simulink library "inp"  (Simulink 7.4)
settings: Solver=ode45  StartTime=0.0  StopTime=10.0  RelTol=1e-3
undefined symbols (not defined in the file): AINP_BrkPedalInterp_X_bar, C_TASK_10MS_S, ENUM_SHIFTER_D, ENUM_SHIFTER_N, ENUM_SHIFTER_P, ENUM_SHIFTER_R, KINP_BonnetCloseVehSpdThre_kph, KINP_EDUCoolantTempFilTm_s, KINP_EDUOilPressureFilTm_s, KINP_EDUOilTempFilTm_s, KINP_EDUSynchDisp_mm, KINP_EDUSynchPosnPWMDC_pct_LowerLimit, KINP_EDUSynchPosnPWMDC_pct_ovrdflg, KINP_EDUSynchPosnPWMDC_pct_ovrdval, KINP_EDUSynchPosnPWMDC_pct_UpperLimit, KINP_ShifterPosConfirmD_s, KINP_ShifterPosConfirmN_s, KINP_ShifterPosConfirmP_s, KINP_ShifterPosConfirmR_s, KINP_SingleAccPedalFltRateLim_pct, KINP_TMSpd2VehSpdSigNeg_rpm, KINP_TMSpd2VehSpdSigPos_rpm, KINP_ValidCheck_EDUSynchPosnPWMDC_dec, KINP_ValidCheck_EDUSynchPosnPWMDC_inc, KINP_ValidCheck_EDUSynchPosnPWMDC_lim, KINP_VehSpdSigKeepThres_kph, KPH2MPS, MIN2SEC, MINP_BrkPedalInterp_pct, MPS2KPH, PI, seat_version_control_block_callbacks, TIRE_RADIUS
libraries: inp_lib x166, hcu_lib x4, simulink x1
(part 7 of 9)

== system inp/INP/INP_20MS/HW_HCU_20ms ==
  BHAL_IN_20ms : Inport
  BSRV_In_ovrdflgs : Inport  Port=2
  BSRV_In_ovrdvals : Inport  Port=3
  Bus Creator : BusCreator  Inputs=2
  Bus Selector18 : BusSelector  OutputSignals=VSRV_EDUOilPressureIn_bar_ovrdval
  Bus Selector20 : BusSelector  OutputSignals=VSRV_EDUOilPressureIn_bar_ovrdflg
  Bus Selector21 : BusSelector  OutputSignals=VHAL_EDUOilPressureIn_bar
  Bus Selector40 : BusSelector  OutputSignals=VHAL_EDUOilPressureValidIn_flg
  Subsys VINP_EDUOilPressure_bar : inp_lib/valid_sat_ovrd  SystemSampleTime=-1  cal_ovrdflg=KINP_EDUOilPressure_bar_ovrdflg  cal_ovrdval=KINP_EDUOilPressure_bar_ovrdval  lim=KINP_ValidCheck_EDUOilPressure_lim  inc=KINP_ValidCheck_EDUOilPressure_inc  dec=KINP_ValidCheck_EDUOilPressure_dec  default=KINP_EDUOilPressureDefault_bar  hi=KINP_EDUOilPressure_bar_UpperLimit  lo=KINP_EDUOilPressure_bar_LowerLimit
  filter : Subsystem
      settings: RTWSystemCode=Inline
  BINP_HW_HCU_20ms : Outport
  wires:
  filter/1(VINP_EDUOilPressure_bar) -> Bus Creator/1  "VINP_EDUOilPressure_bar"
  BHAL_IN_20ms/1 -> Bus Selector21/1, Bus Selector40/1
  BSRV_In_ovrdvals/1 -> [BSRV_In_ovrdvals]
  BSRV_In_ovrdflgs/1 -> [BSRV_In_ovrdflgs]
  Bus Creator/1 -> BINP_HW_HCU_20ms/1  "BINP_HW_HCU_20ms"
  Subsys VINP_EDUOilPressure_bar/1 -> filter/1(VINP_EDUOilPressureRaw_bar)  "VINP_EDUOilPressureRaw_bar"
  Subsys VINP_EDUOilPressure_bar/2 -> Bus Creator/2  "VINP_EDUOilPressureValid_flg"
  [BSRV_In_ovrdvals] -> Bus Selector18/1
  [BSRV_In_ovrdflgs] -> Bus Selector20/1
  Bus Selector21/1 -> Subsys VINP_EDUOilPressure_bar/1  "<VHAL_EDUOilPressureIn_bar>"
  Bus Selector40/1 -> Subsys VINP_EDUOilPressure_bar/2  "<VHAL_EDUOilPressureValidIn_flg>"
  Bus Selector20/1 -> Subsys VINP_EDUOilPressure_bar/3  "<VSRV_EDUOilPressureIn_bar_ovrdflg>"
  Bus Selector18/1 -> Subsys VINP_EDUOilPressure_bar/4  "<VSRV_EDUOilPressureIn_bar_ovrdval>"

== system inp/INP/INP_20MS/Message (15ms) EMS_HSC_FrP03 ==
  BHAL_IN_20ms : Inport
  BSRV_In_ovrdflgs : Inport  Port=2
  BSRV_In_ovrdvals : Inport  Port=3
  VINP_EMSMsgAlive_flg : Inport  Port=4
  Bus Creator : BusCreator  Inputs=5
  Bus Selector1 : BusSelector  OutputSignals=VSRV_AccPedSingleFltIn_flg_ovrdflg
  Bus Selector2 : BusSelector  OutputSignals=VSRV_EMSHSCFrP03Active_flg_ovrdflg
  Bus Selector24 : BusSelector  OutputSignals=VSRV_EngStartReqIn_enum_ovrdval
  Bus Selector26 : BusSelector  OutputSignals=VSRV_EngStartReqIn_enum_ovrdflg
  Bus Selector28 : BusSelector  OutputSignals=VSRV_EngAutoStopInhibitIn_flg_ovrdflg
  Bus Selector29 : BusSelector  OutputSignals=VSRV_EngAutoStopInhibitIn_flg_ovrdval
  Bus Selector3 : BusSelector  OutputSignals=VSRV_EMSHSCFrP03Active_flg_ovrdval
  Bus Selector30 : BusSelector  OutputSignals=VHAL_EngAutoStopInhibitIn_flg
  Bus Selector4 : BusSelector  OutputSignals=VSRV_AccPedSingleFltIn_flg_ovrdval
  Bus Selector5 : BusSelector  OutputSignals=VHAL_AccPedSingleFltIn_flg
  Bus Selector6 : BusSelector  OutputSignals=VHAL_EngStartReqIn_enum
  Bus Selector7 : BusSelector  OutputSignals=VSRV_ACCPedFltIn_flg_ovrdflg
  Bus Selector8 : BusSelector  OutputSignals=VSRV_ACCPedFltIn_flg_ovrdval
  Bus Selector9 : BusSelector  OutputSignals=VHAL_AccPedFltIn_flg
  Subsys VINP_AccPedFlt_flg : inp_lib/msgactv_ovrd  SystemSampleTime=-1  cal_ovrdflg=KINP_AccPedFlt_flg_ovrdflg  cal_ovrdval=KINP_AccPedFlt_flg_ovrdval  default=KINP_AccPedFltDefault_flg
  Subsys VINP_AccPedSingleFlt_flg : inp_lib/msgactv_ovrd  SystemSampleTime=-1  cal_ovrdflg=KINP_AccPedSingleFlt_flg_ovrdflg  cal_ovrdval=KINP_AccPedSingleFlt_flg_ovrdval  default=KINP_AccPedSingleFltDefault_flg
  Subsys VINP_EMSHSCFrP03Active_flg : inp_lib/override  SystemSampleTime=-1  cal_ovrdflg=KINP_EMSHSCFrP03Active_ovrdflg  cal_ovrdval=KINP_EMSHSCFrP03Active_flg_ovrdval
  Subsys VINP_EngAutoStopInhibit_flg : inp_lib/msgactv_ovrd  SystemSampleTime=-1  cal_ovrdflg=KINP_EngAutoStopInhibit_flg_ovrdflg  cal_ovrdval=KINP_EngAutoStopInhibit_flg_ovrdval  default=KINP_EngAutoStopInhibitDefault_flg
  Subsys VINP_EngStartReq_enum : inp_lib/msgactv_sat_ovrd  SystemSampleTime=-1  cal_ovrdflg=KINP_EngStartReq_enum_ovrdflg  cal_ovrdval=KINP_EngStartReq_enum_ovrdval  default=KINP_EngStartReqDefault_enum  hi=255  lo=0
  Terminator{,1..3} (4 alike) : Terminator
  BINP_EMS_HSC_FrP03 : Outport
  wires:
  [BSRV_In_ovrdflgs] -> Bus Selector7/1
  [BSRV_In_ovrdvals] -> Bus Selector8/1
  [BSRV_In_ovrdvals] -> Bus Selector24/1
  [BSRV_In_ovrdflgs] -> Bus Selector26/1
  [BSRV_In_ovrdflgs] -> Bus Selector1/1
  [BSRV_In_ovrdvals] -> Bus Selector4/1
  VINP_EMSMsgAlive_flg/1 -> [VINP_EMSMsgAlive_flg]
  BSRV_In_ovrdflgs/1 -> [BSRV_In_ovrdflgs]
  BSRV_In_ovrdvals/1 -> [BSRV_In_ovrdvals]
  Bus Creator/1 -> BINP_EMS_HSC_FrP03/1  "BINP_EMS_HSC_FrP03"
  BHAL_IN_20ms/1 -> Bus Selector9/1, Bus Selector6/1, Bus Selector5/1, Bus Selector30/1
  [BSRV_In_ovrdflgs] -> Bus Selector28/1
  [BSRV_In_ovrdvals] -> Bus Selector29/1
  [VINP_EMSMsgAlive_flg] -> [MsgAlive_flgs], Subsys VINP_EMSHSCFrP03Active_flg/1
  [BSRV_In_ovrdflgs] -> Bus Selector2/1
  [BSRV_In_ovrdvals] -> Bus Selector3/1
  Bus Selector9/1 -> Subsys VINP_AccPedFlt_flg/1  "<VHAL_AccPedFltIn_flg>"
  Bus Selector7/1 -> Subsys VINP_AccPedFlt_flg/2  "<VSRV_ACCPedFltIn_flg_ovrdflg>"
  Bus Selector8/1 -> Subsys VINP_AccPedFlt_flg/3  "<VSRV_ACCPedFltIn_flg_ovrdval>"
  [MsgAlive_flgs] -> Subsys VINP_AccPedFlt_flg/4
  Subsys VINP_AccPedFlt_flg/1 -> Bus Creator/3  "VINP_AccPedFlt_flg"
  Subsys VINP_AccPedFlt_flg/2 -> Terminator/1
  Bus Selector5/1 -> Subsys VINP_AccPedSingleFlt_flg/1  "<VHAL_AccPedSingleFltIn_flg>"
  Bus Selector1/1 -> Subsys VINP_AccPedSingleFlt_flg/2  "<VSRV_AccPedSingleFltIn_flg_ovrdflg>"
  Bus Selector4/1 -> Subsys VINP_AccPedSingleFlt_flg/3  "<VSRV_AccPedSingleFltIn_flg_ovrdval>"
  [MsgAlive_flgs] -> Subsys VINP_AccPedSingleFlt_flg/4
  Subsys VINP_AccPedSingleFlt_flg/1 -> Bus Creator/2  "VINP_AccPedSingleFlt_flg"
  Subsys VINP_AccPedSingleFlt_flg/2 -> Terminator1/1
  Bus Selector2/1 -> Subsys VINP_EMSHSCFrP03Active_flg/2  "<VSRV_EMSHSCFrP03Active_flg_ovrdflg>"
  Bus Selector3/1 -> Subsys VINP_EMSHSCFrP03Active_flg/3  "<VSRV_EMSHSCFrP03Active_flg_ovrdval>"
  Subsys VINP_EMSHSCFrP03Active_flg/1 -> Bus Creator/5  "VINP_EMSHSCFrP03Active_flg"
  Bus Selector30/1 -> Subsys VINP_EngAutoStopInhibit_flg/1  "<VHAL_EngAutoStopInhibitIn_flg>"
  Bus Selector28/1 -> Subsys VINP_EngAutoStopInhibit_flg/2  "<VSRV_EngAutoStopInhibitIn_flg_ovrdflg>"
  Bus Selector29/1 -> Subsys VINP_EngAutoStopInhibit_flg/3  "<VSRV_EngAutoStopInhibitIn_flg_ovrdval>"
  [MsgAlive_flgs] -> Subsys VINP_EngAutoStopInhibit_flg/4
  Subsys VINP_EngAutoStopInhibit_flg/1 -> Bus Creator/1  "VINP_EngAutoStopInhibit_flg"
  Subsys VINP_EngAutoStopInhibit_flg/2 -> Terminator2/1
  Bus Selector6/1 -> Subsys VINP_EngStartReq_enum/1  "<VHAL_EngStartReqIn_enum>"
  Bus Selector26/1 -> Subsys VINP_EngStartReq_enum/2  "<VSRV_EngStartReqIn_enum_ovrdflg>"
  Bus Selector24/1 -> Subsys VINP_EngStartReq_enum/3  "<VSRV_EngStartReqIn_enum_ovrdval>"
  [MsgAlive_flgs] -> Subsys VINP_EngStartReq_enum/4
  Subsys VINP_EngStartReq_enum/1 -> Bus Creator/4  "VINP_EngStartReq_enum"
  Subsys VINP_EngStartReq_enum/2 -> Terminator3/1

== system inp/INP/INP_20MS/Message (20ms) BMS_HSC2_FrP03 ==
  BHAL_IN_20ms : Inport
  BSRV_In_ovrdflgs : Inport  Port=2
  BSRV_In_ovrdvals : Inport  Port=3
  VINP_BMSMsgAlive_flg : Inport  Port=4
  Bus Creator : BusCreator  Inputs=6
  Bus Selector1 : BusSelector  OutputSignals=VSRV_HVBattEnergyAvailIn_kWh_ovrdval
  Bus Selector10 : BusSelector  OutputSignals=VSRV_HVBattBalanceReqIn_flg_ovrdval
  Bus Selector11 : BusSelector  OutputSignals=VHAL_HVBattBalanceReqIn_flg
  Bus Selector12 : BusSelector  OutputSignals=VSRV_HVBattFltLampOnReqIn_flg_ovrdval
  Bus Selector13 : BusSelector  OutputSignals=VHAL_HVBattFltLampOnReqIn_flg
  Bus Selector14 : BusSelector  OutputSignals=VSRV_HVBattFltLampOnReqIn_flg_ovrdflg
  Bus Selector2 : BusSelector  OutputSignals=VSRV_BMSHSC2FrP03Active_flg_ovrdflg
  Bus Selector3 : BusSelector  OutputSignals=VSRV_BMSHSC2FrP03Active_flg_ovrdval
  Bus Selector38 : BusSelector  OutputSignals=VSRV_HVBattChargeCurrMaxIn_A_ovrdval
  Bus Selector4 : BusSelector  OutputSignals=VHAL_HVBattEnergyAvailIn_kWh
  Bus Selector40 : BusSelector  OutputSignals=VHAL_HVBattChargeCurrMaxIn_A
  Bus Selector42 : BusSelector  OutputSignals=VSRV_HVBattChargeCurrMaxIn_A_ovrdflg
  Bus Selector43 : BusSelector  OutputSignals=VSRV_HVBattDischargeCurrMaxIn_A_ovrdval
  Bus Selector44 : BusSelector  OutputSignals=VHAL_HVBattDischargeCurrMaxIn_A
  Bus Selector46 : BusSelector  OutputSignals=VSRV_HVBattDischargeCurrMaxIn_A_ovrdflg
  Bus Selector5 : BusSelector  OutputSignals=VHAL_HVBattChargeCurrMaxValidIn_flg
  Bus Selector6 : BusSelector  OutputSignals=VHAL_HVBattDischargeCurrMaxValidIn_flg
  Bus Selector7 : BusSelector  OutputSignals=VSRV_HVBattEnergyAvailIn_kWh_ovrdflg
  Bus Selector8 : BusSelector  OutputSignals=VHAL_HVBattEnergyAvailValidIn_flg
  Bus Selector9 : BusSelector  OutputSignals=VSRV_HVBattBalanceReqIn_flg_ovrdflg
  Subsys VINP_BMSHSC2FrP03Active_flg : inp_lib/override  SystemSampleTime=-1  cal_ovrdflg=KINP_BMSHSC2FrP03Active_ovrdflg  cal_ovrdval=KINP_BMSHSC2FrP03Active_flg_ovrdval
  Subsys VINP_HVBattBalanceReq_flg : inp_lib/msgactv_ovrd  SystemSampleTime=-1  cal_ovrdflg=KINP_HVBattBalanceReq_flg_ovrdflg  cal_ovrdval=KINP_HVBattBalanceReq_flg_ovrdval  default=KINP_HVBattBalanceReqDefault_flg
  Subsys VINP_HVBattChargeCurrMax_A : inp_lib/valid_msgactv_sat_ovrd  SystemSampleTime=-1  cal_ovrdflg=KINP_HVBattChargeCurrMax_A_ovrdflg  cal_ovrdval=KINP_HVBattChargeCurrMax_A_ovrdval  lim=KINP_ValidCheck_HVBattChargeCurrMax_lim  inc=KINP_ValidCheck_HVBattChargeCurrMax_inc  dec=KINP_ValidCheck_HVBattChargeCurrMax_dec  default=KINP_HVBattChargeCurrMaxDefault_A  hi=KINP_HVBattChargeCurrMax_A_Max  lo=KINP_HVBattChargeCurrMax_A_Min
  Subsys VINP_HVBattDisChargeCurrMax_A : inp_lib/valid_msgactv_sat_ovrd  SystemSampleTime=-1  cal_ovrdflg=KINP_HVBattDisChargeCurrMax_A_ovrdflg  cal_ovrdval=KINP_HVBattDisChargeCurrMax_A_ovrdval  lim=KINP_ValidCheck_HVBattDisChargeCurrMax_lim  inc=KINP_ValidCheck_HVBattDisChargeCurrMax_inc  dec=KINP_ValidCheck_HVBattDisChargeCurrMax_dec  default=KINP_HVBattDisChargeCurrMaxDefault_A  hi=KINP_HVBattDisChargeCurrMax_A_Max  lo=KINP_HVBattDisChargeCurrMax_A_Min
  Subsys VINP_HVBattEnergyAvail_kWh : inp_lib/valid_msgactv_sat_ovrd  SystemSampleTime=-1  cal_ovrdflg=KINP_HVBattEnergyAvail_kWh_ovrdflg  cal_ovrdval=KINP_HVBattEnergyAvail_kWh_ovrdval  lim=KINP_ValidCheck_HVBattEnergyAvail_lim  inc=KINP_ValidCheck_HVBattEnergyAvail_inc  dec=KINP_ValidCheck_HVBattEnergyAvail_dec  default=KINP_HVBattEnergyAvailDefault_kWh  hi=KINP_HVBattEnergyAvail_kWh_Max  lo=KINP_HVBattEnergyAvail_kWh_Min
  Subsys VINP_HVBattFltLampOnReq_flg : inp_lib/msgactv_ovrd  SystemSampleTime=-1  cal_ovrdflg=KINP_HVBattFltLampOnReq_flg_ovrdflg  cal_ovrdval=KINP_HVBattFltLampOnReq_flg_ovrdval  default=KINP_HVBattFltLampOnReqDefault_flg
  Terminator{,1..4} (5 alike) : Terminator
  BINP_BMS_HSC2_FrP03 : Outport
  wires:
  [BSRV_In_ovrdflgs] -> Bus Selector14/1
  [BSRV_In_ovrdvals] -> Bus Selector12/1
  [BSRV_In_ovrdflgs] -> Bus Selector9/1
  [BSRV_In_ovrdvals] -> Bus Selector10/1
  [BSRV_In_ovrdvals] -> Bus Selector1/1
  [BSRV_In_ovrdflgs] -> Bus Selector7/1
  VINP_BMSMsgAlive_flg/1 -> [VINP_BMSMsgAlive_flg]
  BSRV_In_ovrdflgs/1 -> [BSRV_In_ovrdflgs]
  BSRV_In_ovrdvals/1 -> [BSRV_In_ovrdvals]
  BHAL_IN_20ms/1 -> Bus Selector6/1, Bus Selector44/1, Bus Selector13/1, Bus Selector11/1, Bus Selector8/1, Bus Selector4/1, Bus Selector5/1, Bus Selector40/1
  [BSRV_In_ovrdflgs] -> Bus Selector2/1
  [BSRV_In_ovrdvals] -> Bus Selector3/1
  [BSRV_In_ovrdvals] -> Bus Selector38/1
  [BSRV_In_ovrdflgs] -> Bus Selector42/1
  [BSRV_In_ovrdvals] -> Bus Selector43/1
  [BSRV_In_ovrdflgs] -> Bus Selector46/1
  Bus Creator/1 -> BINP_BMS_HSC2_FrP03/1  "BINP_BMS_HSC2_FrP03"
  Bus Selector2/1 -> Subsys VINP_BMSHSC2FrP03Active_flg/2  "<VSRV_BMSHSC2FrP03Active_flg_ovrdflg>"
  Bus Selector3/1 -> Subsys VINP_BMSHSC2FrP03Active_flg/3  "<VSRV_BMSHSC2FrP03Active_flg_ovrdval>"
  Subsys VINP_BMSHSC2FrP03Active_flg/1 -> Bus Creator/6  "VINP_BMSHSC2FrP03Active_flg"
  Bus Selector11/1 -> Subsys VINP_HVBattBalanceReq_flg/1  "<VHAL_HVBattBalanceReqIn_flg>"
  Bus Selector9/1 -> Subsys VINP_HVBattBalanceReq_flg/2  "<VSRV_HVBattBalanceReqIn_flg_ovrdflg>"
  Bus Selector10/1 -> Subsys VINP_HVBattBalanceReq_flg/3  "<VSRV_HVBattBalanceReqIn_flg_ovrdval>"
  [MsgAlive_flgs] -> Subsys VINP_HVBattBalanceReq_flg/4
  Subsys VINP_HVBattBalanceReq_flg/1 -> Bus Creator/3  "VINP_HVBattBalanceReq_flg"
  Subsys VINP_HVBattBalanceReq_flg/2 -> Terminator/1
  Bus Selector40/1 -> Subsys VINP_HVBattChargeCurrMax_A/1  "<VHAL_HVBattChargeCurrMaxIn_A>"
  Bus Selector5/1 -> Subsys VINP_HVBattChargeCurrMax_A/2  "<VHAL_HVBattChargeCurrMaxValidIn_flg>"
  Bus Selector42/1 -> Subsys VINP_HVBattChargeCurrMax_A/3  "<VSRV_HVBattChargeCurrMaxIn_A_ovrdflg>"
  Bus Selector38/1 -> Subsys VINP_HVBattChargeCurrMax_A/4  "<VSRV_HVBattChargeCurrMaxIn_A_ovrdval>"
  [MsgAlive_flgs] -> Subsys VINP_HVBattChargeCurrMax_A/5
  Subsys VINP_HVBattChargeCurrMax_A/1 -> Bus Creator/1  "VINP_HVBattChargeCurrMax_A"
  Subsys VINP_HVBattChargeCurrMax_A/2 -> Terminator1/1
  Bus Selector44/1 -> Subsys VINP_HVBattDisChargeCurrMax_A/1  "<VHAL_HVBattDischargeCurrMaxIn_A>"
  Bus Selector6/1 -> Subsys VINP_HVBattDisChargeCurrMax_A/2  "<VHAL_HVBattDischargeCurrMaxValidIn_flg>"
  Bus Selector46/1 -> Subsys VINP_HVBattDisChargeCurrMax_A/3  "<VSRV_HVBattDischargeCurrMaxIn_A_ovrdflg>"
  Bus Selector43/1 -> Subsys VINP_HVBattDisChargeCurrMax_A/4  "<VSRV_HVBattDischargeCurrMaxIn_A_ovrdval>"
  [MsgAlive_flgs] -> Subsys VINP_HVBattDisChargeCurrMax_A/5
  Subsys VINP_HVBattDisChargeCurrMax_A/1 -> Bus Creator/5  "VINP_HVBattDisChargeCurrMax_A"
  Subsys VINP_HVBattDisChargeCurrMax_A/2 -> Terminator2/1
  Bus Selector4/1 -> Subsys VINP_HVBattEnergyAvail_kWh/1  "<VHAL_HVBattEnergyAvailIn_kWh>"
  Bus Selector8/1 -> Subsys VINP_HVBattEnergyAvail_kWh/2  "<VHAL_HVBattEnergyAvailValidIn_flg>"
  Bus Selector7/1 -> Subsys VINP_HVBattEnergyAvail_kWh/3  "<VSRV_HVBattEnergyAvailIn_kWh_ovrdflg>"
  Bus Selector1/1 -> Subsys VINP_HVBattEnergyAvail_kWh/4  "<VSRV_HVBattEnergyAvailIn_kWh_ovrdval>"
  [MsgAlive_flgs] -> Subsys VINP_HVBattEnergyAvail_kWh/5
  Subsys VINP_HVBattEnergyAvail_kWh/1 -> Bus Creator/2  "VINP_HVBattEnergyAvail_kWh"
  Subsys VINP_HVBattEnergyAvail_kWh/2 -> Terminator3/1
  Bus Selector13/1 -> Subsys VINP_HVBattFltLampOnReq_flg/1  "<VHAL_HVBattFltLampOnReqIn_flg>"
  Bus Selector14/1 -> Subsys VINP_HVBattFltLampOnReq_flg/2  "<VSRV_HVBattFltLampOnReqIn_flg_ovrdflg>"
  Bus Selector12/1 -> Subsys VINP_HVBattFltLampOnReq_flg/3  "<VSRV_HVBattFltLampOnReqIn_flg_ovrdval>"
  [MsgAlive_flgs] -> Subsys VINP_HVBattFltLampOnReq_flg/4
  Subsys VINP_HVBattFltLampOnReq_flg/1 -> Bus Creator/4  "VINP_HVBattFltLampOnReq_flg"
  Subsys VINP_HVBattFltLampOnReq_flg/2 -> Terminator4/1
  [VINP_BMSMsgAlive_flg] -> Subsys VINP_BMSHSC2FrP03Active_flg/1, [MsgAlive_flgs]  "VINP_BMSMsgAlive_flg"

== system inp/INP/INP_20MS/Message (20ms) BMS_HSC2_FrP09 ==
  BHAL_IN_20ms : Inport
  BSRV_In_ovrdflgs : Inport  Port=2
  BSRV_In_ovrdvals : Inport  Port=3
  VINP_BMSMsgAlive_flg : Inport  Port=4
  Bus Creator : BusCreator  Inputs=8
  Bus Selector1 : BusSelector  OutputSignals=VHAL_BMSPeakChrgPwrValidIn_flg
  Bus Selector10 : BusSelector  OutputSignals=VHAL_BMSDchaBufferIn_pct
  Bus Selector11 : BusSelector  OutputSignals=VHAL_HVBattPwrAvailChargeValidIn_flg
  Bus Selector113 : BusSelector  OutputSignals=VSRV_HVBattPwrAvailChargeIn_kW_ovrdflg
  Bus Selector114 : BusSelector  OutputSignals=VSRV_HVBattPwrAvailChargeIn_kW_ovrdval
  Bus Selector115 : BusSelector  OutputSignals=VSRV_HVBattPwrAvailDischargeIn_kW_ovrdflg
  Bus Selector116 : BusSelector  OutputSignals=VSRV_HVBattPwrAvailDischargeIn_kW_ovrdval
  Bus Selector117 : BusSelector  OutputSignals=VHAL_HVBattPwrAvailDischargeIn_kW
  Bus Selector118 : BusSelector  OutputSignals=VHAL_BMSChrgBufferIn_pct
  Bus Selector12 : BusSelector  OutputSignals=VHAL_HVBattPwrAvailDischargeValidIn_flg
  Bus Selector120 : BusSelector  OutputSignals=VSRV_BMSChrgBufferIn_pct_ovrdflg
  Bus Selector13 : BusSelector  OutputSignals=VSRV_BMSDchaBufferIn_pct_ovrdflg
  Bus Selector14 : BusSelector  OutputSignals=VSRV_BMSDchaBufferIn_pct_ovrdval
  Bus Selector15 : BusSelector  OutputSignals=VHAL_BMSDchaBufferValidIn_flg
  Bus Selector2 : BusSelector  OutputSignals=VSRV_BMSPeakChrgPwrIn_kW_ovrdflg
  Bus Selector26 : BusSelector  OutputSignals=VHAL_HVBattPwrAvailChargeIn_kW
  Bus Selector28 : BusSelector  OutputSignals=VSRV_BMSChrgBufferIn_pct_ovrdval
  Bus Selector3 : BusSelector  OutputSignals=VSRV_BMSPeakChrgPwrIn_kW_ovrdval
  Bus Selector4 : BusSelector  OutputSignals=VSRV_BMSPeakDchaPwrIn_kW_ovrdflg
  Bus Selector5 : BusSelector  OutputSignals=VSRV_BMSPeakDchaPwrIn_kW_ovrdval
  Bus Selector6 : BusSelector  OutputSignals=VHAL_BMSPeakDchaPwrIn_kW
  Bus Selector7 : BusSelector  OutputSignals=VHAL_BMSPeakDchaPwrValidIn_flg
  Bus Selector8 : BusSelector  OutputSignals=VHAL_BMSPeakChrgPwrIn_kW
  Bus Selector9 : BusSelector  OutputSignals=VHAL_BMSChrgBufferValidIn_flg
  Subsys VINP_BMSChrgBuffer_pct : inp_lib/valid_msgactv_sat_ovrd  SystemSampleTime=-1  cal_ovrdflg=KINP_BMSChrgBuffer_pct_ovrdflg  cal_ovrdval=KINP_BMSChrgBuffer_pct_ovrdval  lim=KINP_ValidCheck_BMSChrgBuffer_lim  inc=KINP_ValidCheck_BMSChrgBuffer_inc  dec=KINP_ValidCheck_BMSChrgBuffer_dec  default=KINP_BMSChrgBufferDefault_pct  hi=KINP_BMSChrgBuffer_pct_Max  lo=KINP_BMSChrgBuffer_pct_Min
  Subsys VINP_BMSDchaBuffer_pct : inp_lib/valid_msgactv_sat_ovrd  SystemSampleTime=-1  cal_ovrdflg=KINP_BMSDchaBuffer_pct_ovrdflg  cal_ovrdval=KINP_BMSDchaBuffer_pct_ovrdval  lim=KINP_ValidCheck_BMSDchaBuffer_lim  inc=KINP_ValidCheck_BMSDchaBuffer_inc  dec=KINP_ValidCheck_BMSDchaBuffer_dec  default=KINP_BMSDchaBufferDefault_pct  hi=KINP_BMSDchaBuffer_pct_Max  lo=KINP_BMSDchaBuffer_pct_Min
  Subsys VINP_BMSPeakChrgPwr_kW : inp_lib/valid_msgactv_sat_ovrd  SystemSampleTime=-1  cal_ovrdflg=KINP_BMSPeakChrgPwr_kW_ovrdflg  cal_ovrdval=KINP_BMSPeakChrgPwr_kW_ovrdval  lim=KINP_ValidCheck_BMSPeakChrgPwr_lim  inc=KINP_ValidCheck_BMSPeakChrgPwr_inc  dec=KINP_ValidCheck_BMSPeakChrgPwr_dec  default=KINP_BMSPeakChrgPwrDefault_kW  hi=KINP_BMSPeakChrgPwr_kW_Max  lo=KINP_BMSPeakChrgPwr_kW_Min
  Subsys VINP_BMSPeakDchaPwr_kW : inp_lib/valid_msgactv_sat_ovrd  SystemSampleTime=-1  cal_ovrdflg=KINP_BMSPeakDchaPwr_kW_ovrdflg  cal_ovrdval=KINP_BMSPeakDchaPwr_kW_ovrdval  lim=KINP_ValidCheck_BMSPeakDchaPwr_lim  inc=KINP_ValidCheck_BMSPeakDchaPwr_inc  dec=KINP_ValidCheck_BMSPeakDchaPwr_dec  default=KINP_BMSPeakDchaPwrDefault_kW  hi=KINP_BMSPeakDchaPwr_kW_Max  lo=KINP_BMSPeakDchaPwr_kW_Min
  Subsys VINP_HVBattPwrAvailCharge_kW : inp_lib/valid_msgactv_sat_ovrd  SystemSampleTime=-1  cal_ovrdflg=KINP_HVBattPwrAvailCharge_kW_ovrdflg  cal_ovrdval=KINP_HVBattPwrAvailCharge_kW_ovrdval  lim=KINP_ValidCheck_HVBattPwrAvailCharge_lim  inc=KINP_ValidCheck_HVBattPwrAvailCharge_inc  dec=KINP_ValidCheck_HVBattPwrAvailCharge_dec  default=KINP_HVBattPwrAvailChargeDefault_kW  hi=KINP_HVBattPwrAvailCharge_kW_Max  lo=KINP_HVBattPwrAvailCharge_kW_Min
  Subsys VINP_HVBattPwrAvailDischarge_kW : inp_lib/valid_msgactv_sat_ovrd  SystemSampleTime=-1  cal_ovrdflg=KINP_HVBattPwrAvailDischarge_kW_ovrdflg  cal_ovrdval=KINP_HVBattPwrAvailDischarge_kW_ovrdval  lim=KINP_ValidCheck_HVBattPwrAvailDischarge_lim  inc=KINP_ValidCheck_HVBattPwrAvailDischarge_inc  dec=KINP_ValidCheck_HVBattPwrAvailDischarge_dec  default=KINP_HVBattPwrAvailDischargeDefault_kW  hi=KINP_HVBattPwrAvailDischarge_kW_Max  lo=KINP_HVBattPwrAvailDischarge_kW_Min
  Terminator{3..6} (4 alike) : Terminator
  BINP_BMS_HSC2_FrP09 : Outport
  wires:
  Subsys VINP_BMSDchaBuffer_pct/1 -> Bus Creator/8  "VINP_BMSDchaBuffer_pct"
  Subsys VINP_BMSChrgBuffer_pct/1 -> Bus Creator/7  "VINP_BMSChrgBuffer_pct"
  Subsys VINP_BMSPeakDchaPwr_kW/1 -> Bus Creator/5  "VINP_BMSPeakDchaPwr_kW"
  [BSRV_In_ovrdflgs] -> Bus Selector13/1
  [BSRV_In_ovrdvals] -> Bus Selector14/1
  Bus Selector10/1 -> Subsys VINP_BMSDchaBuffer_pct/1  "<VHAL_BMSDchaBufferIn_pct>"
  Bus Selector15/1 -> Subsys VINP_BMSDchaBuffer_pct/2  "<VHAL_BMSDchaBufferValidIn_flg>"
  Bus Selector13/1 -> Subsys VINP_BMSDchaBuffer_pct/3  "<VSRV_BMSDchaBufferIn_pct_ovrdflg>"
  Bus Selector14/1 -> Subsys VINP_BMSDchaBuffer_pct/4  "<VSRV_BMSDchaBufferIn_pct_ovrdval>"
  [MsgAlive_flgs] -> Subsys VINP_BMSDchaBuffer_pct/5
  Subsys VINP_BMSDchaBuffer_pct/2 -> Terminator4/1
  [BSRV_In_ovrdflgs] -> Bus Selector120/1
  [BSRV_In_ovrdvals] -> Bus Selector28/1
  Bus Selector118/1 -> Subsys VINP_BMSChrgBuffer_pct/1  "<VHAL_BMSChrgBufferIn_pct>"
  Bus Selector9/1 -> Subsys VINP_BMSChrgBuffer_pct/2  "<VHAL_BMSChrgBufferValidIn_flg>"
  Bus Selector120/1 -> Subsys VINP_BMSChrgBuffer_pct/3  "<VSRV_BMSChrgBufferIn_pct_ovrdflg>"
  Bus Selector28/1 -> Subsys VINP_BMSChrgBuffer_pct/4  "<VSRV_BMSChrgBufferIn_pct_ovrdval>"
  [MsgAlive_flgs] -> Subsys VINP_BMSChrgBuffer_pct/5
  Subsys VINP_BMSChrgBuffer_pct/2 -> Terminator3/1
  [BSRV_In_ovrdflgs] -> Bus Selector2/1
  [BSRV_In_ovrdvals] -> Bus Selector3/1
  [BSRV_In_ovrdflgs] -> Bus Selector4/1
  [BSRV_In_ovrdvals] -> Bus Selector5/1
  Bus Selector8/1 -> Subsys VINP_BMSPeakChrgPwr_kW/1  "<VHAL_BMSPeakChrgPwrIn_kW>"
  Bus Selector1/1 -> Subsys VINP_BMSPeakChrgPwr_kW/2  "<VHAL_BMSPeakChrgPwrValidIn_flg>"
  Bus Selector2/1 -> Subsys VINP_BMSPeakChrgPwr_kW/3  "<VSRV_BMSPeakChrgPwrIn_kW_ovrdflg>"
  Bus Selector3/1 -> Subsys VINP_BMSPeakChrgPwr_kW/4  "<VSRV_BMSPeakChrgPwrIn_kW_ovrdval>"
  [MsgAlive_flgs] -> Subsys VINP_BMSPeakChrgPwr_kW/5
  Subsys VINP_BMSPeakChrgPwr_kW/1 -> Bus Creator/3  "VINP_BMSPeakChrgPwr_kW"
  Subsys VINP_BMSPeakChrgPwr_kW/2 -> Bus Creator/4  "VINP_BMSPeakChrgPwrVld_flg"
  Bus Selector6/1 -> Subsys VINP_BMSPeakDchaPwr_kW/1  "<VHAL_BMSPeakDchaPwrIn_kW>"
  Bus Selector7/1 -> Subsys VINP_BMSPeakDchaPwr_kW/2  "<VHAL_BMSPeakDchaPwrValidIn_flg>"
  Bus Selector4/1 -> Subsys VINP_BMSPeakDchaPwr_kW/3  "<VSRV_BMSPeakDchaPwrIn_kW_ovrdflg>"
  Bus Selector5/1 -> Subsys VINP_BMSPeakDchaPwr_kW/4  "<VSRV_BMSPeakDchaPwrIn_kW_ovrdval>"
  [MsgAlive_flgs] -> Subsys VINP_BMSPeakDchaPwr_kW/5
  Subsys VINP_BMSPeakDchaPwr_kW/2 -> Bus Creator/6  "VINP_BMSPeakDchaPwrVld_flg"
  Subsys VINP_HVBattPwrAvailDischarge_kW/1 -> Bus Creator/2  "VINP_HVBattPwrAvailDischarge_kW"
  [BSRV_In_ovrdflgs] -> Bus Selector113/1
  [BSRV_In_ovrdvals] -> Bus Selector114/1
  [BSRV_In_ovrdflgs] -> Bus Selector115/1
  [BSRV_In_ovrdvals] -> Bus Selector116/1
  Bus Selector26/1 -> Subsys VINP_HVBattPwrAvailCharge_kW/1  "<VHAL_HVBattPwrAvailChargeIn_kW>"
  Bus Selector11/1 -> Subsys VINP_HVBattPwrAvailCharge_kW/2  "<VHAL_HVBattPwrAvailChargeValidIn_flg>"
  Bus Selector113/1 -> Subsys VINP_HVBattPwrAvailCharge_kW/3  "<VSRV_HVBattPwrAvailChargeIn_kW_ovrdflg>"
  Bus Selector114/1 -> Subsys VINP_HVBattPwrAvailCharge_kW/4  "<VSRV_HVBattPwrAvailChargeIn_kW_ovrdval>"
  [MsgAlive_flgs] -> Subsys VINP_HVBattPwrAvailCharge_kW/5
  Subsys VINP_HVBattPwrAvailCharge_kW/1 -> Bus Creator/1  "VINP_HVBattPwrAvailCharge_kW"
  Subsys VINP_HVBattPwrAvailCharge_kW/2 -> Terminator5/1
  Bus Selector117/1 -> Subsys VINP_HVBattPwrAvailDischarge_kW/1  "<VHAL_HVBattPwrAvailDischargeIn_kW>"
  Bus Selector12/1 -> Subsys VINP_HVBattPwrAvailDischarge_kW/2  "<VHAL_HVBattPwrAvailDischargeValidIn_flg>"
  Bus Selector115/1 -> Subsys VINP_HVBattPwrAvailDischarge_kW/3  "<VSRV_HVBattPwrAvailDischargeIn_kW_ovrdflg>"
  Bus Selector116/1 -> Subsys VINP_HVBattPwrAvailDischarge_kW/4  "<VSRV_HVBattPwrAvailDischargeIn_kW_ovrdval>"
  [MsgAlive_flgs] -> Subsys VINP_HVBattPwrAvailDischarge_kW/5
  Subsys VINP_HVBattPwrAvailDischarge_kW/2 -> Terminator6/1
  VINP_BMSMsgAlive_flg/1 -> [MsgAlive_flgs]
  BSRV_In_ovrdflgs/1 -> [BSRV_In_ovrdflgs]
  BSRV_In_ovrdvals/1 -> [BSRV_In_ovrdvals]
  BHAL_IN_20ms/1 -> Bus Selector1/1, Bus Selector15/1, Bus Selector10/1, Bus Selector9/1, Bus Selector118/1, Bus Selector7/1, Bus Selector6/1, Bus Selector8/1, Bus Selector12/1, Bus Selector117/1, Bus Selector11/1, Bus Selector26/1
  Bus Creator/1 -> BINP_BMS_HSC2_FrP09/1  "BINP_BMS_HSC2_FrP09"

== system inp/INP/INP_20MS/Message (20ms) DSC_HSC_FrP04 ==
  BHAL_IN_20ms : Inport
  BSRV_In_ovrdflgs : Inport  Port=2
  BSRV_In_ovrdvals : Inport  Port=3
  VINP_DSCMsgAlive_flg : Inport  Port=4
  Bus Creator : BusCreator
  Bus Selector11 : BusSelector  OutputSignals=VHAL_ESPRegenFaultIn_flg
  Bus Selector13 : BusSelector  OutputSignals=VSRV_ESPRegenFaultIn_flg_ovrdflg
  Bus Selector14 : BusSelector  OutputSignals=VSRV_ESPRegenFaultIn_flg_ovrdval
  Bus Selector15 : BusSelector  OutputSignals=VSRV_ESPRegenTargetIn_Nm_ovrdval
  Bus Selector16 : BusSelector  OutputSignals=VHAL_ESPRegenTargetAtWheelIn_Nm
  Bus Selector18 : BusSelector  OutputSignals=VSRV_ESPRegenTargetIn_Nm_ovrdflg
  Bus Selector2 : BusSelector  OutputSignals=VSRV_DSCHSCFrP04Active_flg_ovrdflg
  Bus Selector3 : BusSelector  OutputSignals=VSRV_DSCHSCFrP04Active_flg_ovrdval
  Bus Selector4 : BusSelector  OutputSignals=VHAL_ESPRegenTargetValidIn_flg
  Bus Selector55 : BusSelector  OutputSignals=VHAL_BrkVacPumpStateIn_enum
  Bus Selector57 : BusSelector  OutputSignals=VSRV_BrkVacPumpStateIn_enum_ovrdflg
  Bus Selector58 : BusSelector  OutputSignals=VSRV_BrkVacPumpStateIn_enum_ovrdval
  Subsys VINP_BrkVacPumpState_enum : inp_lib/msgactv_sat_ovrd  SystemSampleTime=-1  cal_ovrdflg=KINP_BrkVacPumpState_enum_ovrdflg  cal_ovrdval=KINP_BrkVacPumpState_enum_ovrdval  default=KINP_BrkVacPumpStateDefault_enum  hi=KINP_BrkVacPumpState_enum_Max  lo=KINP_BrkVacPumpState_enum_Min
  Subsys VINP_DSCHSCFrP04Active_flg : inp_lib/override  SystemSampleTime=-1  cal_ovrdflg=KINP_DSCHSCFrP04Active_ovrdflg  cal_ovrdval=KINP_DSCHSCFrP04Active_flg_ovrdval
  Subsys VINP_ESPRegenFault_flg : inp_lib/msgactv_ovrd  SystemSampleTime=-1  cal_ovrdflg=KINP_ESPRegenFault_flg_ovrdflg  cal_ovrdval=KINP_ESPRegenFault_flg_ovrdval  default=KINP_ESPRegenFaultDefault_flg
  Subsys VINP_ESPRegenTargetAtWheel_Nm : inp_lib/valid_msgactv_sat_ovrd  SystemSampleTime=-1  cal_ovrdflg=KINP_ESPRegenTargetAtWheel_Nm_ovrdflg  cal_ovrdval=KINP_ESPRegenTargetAtWheel_Nm_ovrdval  lim=KINP_ValidCheck_ESPRegenTargetAtWheel_lim  inc=KINP_ValidCheck_ESPRegenTargetAtWheel_inc  dec=KINP_ValidCheck_ESPRegenTargetAtWheel_dec  default=KINP_ESPRegenTargetAtWheelDefault_Nm  hi=KINP_ESPRegenTargetAtWheel_Nm_Max  lo=KINP_ESPRegenTargetAtWheel_Nm_Min
  Terminator : Terminator
  Terminator1 : Terminator
  Terminator2 : Terminator
  BINP_DSC_HSC_FrP04 : Outport
  wires:
  [BSRV_In_ovrdflgs] -> Bus Selector57/1
  [BSRV_In_ovrdvals] -> Bus Selector58/1
  [VINP_DSCMsgAlive_flg] -> [MsgAlive_flgs], Subsys VINP_DSCHSCFrP04Active_flg/1
  [BSRV_In_ovrdflgs] -> Bus Selector2/1
  [BSRV_In_ovrdvals] -> Bus Selector3/1
  [BSRV_In_ovrdflgs] -> Bus Selector18/1
  [BSRV_In_ovrdvals] -> Bus Selector15/1
  BHAL_IN_20ms/1 -> Bus Selector55/1, Bus Selector11/1, Bus Selector4/1, Bus Selector16/1
  [BSRV_In_ovrdvals] -> Bus Selector14/1
  [BSRV_In_ovrdflgs] -> Bus Selector13/1
  Bus Creator/1 -> BINP_DSC_HSC_FrP04/1  "BINP_DSC_HSC_FrP04"
  BSRV_In_ovrdvals/1 -> [BSRV_In_ovrdvals]
  BSRV_In_ovrdflgs/1 -> [BSRV_In_ovrdflgs]
  VINP_DSCMsgAlive_flg/1 -> [VINP_DSCMsgAlive_flg]
  Bus Selector55/1 -> Subsys VINP_BrkVacPumpState_enum/1  "<VHAL_BrkVacPumpStateIn_enum>"
  Bus Selector57/1 -> Subsys VINP_BrkVacPumpState_enum/2  "<VSRV_BrkVacPumpStateIn_enum_ovrdflg>"
  Bus Selector58/1 -> Subsys VINP_BrkVacPumpState_enum/3  "<VSRV_BrkVacPumpStateIn_enum_ovrdval>"
  [MsgAlive_flgs] -> Subsys VINP_BrkVacPumpState_enum/4
  Subsys VINP_BrkVacPumpState_enum/1 -> Bus Creator/1  "VINP_BrkVacPumpState_enum"
  Subsys VINP_BrkVacPumpState_enum/2 -> Terminator/1
  Bus Selector2/1 -> Subsys VINP_DSCHSCFrP04Active_flg/2  "<VSRV_DSCHSCFrP04Active_flg_ovrdflg>"
  Bus Selector3/1 -> Subsys VINP_DSCHSCFrP04Active_flg/3  "<VSRV_DSCHSCFrP04Active_flg_ovrdval>"
  Subsys VINP_DSCHSCFrP04Active_flg/1 -> Bus Creator/4  "VINP_DSCHSCFrP04Active_flg"
  Bus Selector11/1 -> Subsys VINP_ESPRegenFault_flg/1  "<VHAL_ESPRegenFaultIn_flg>"
  Bus Selector13/1 -> Subsys VINP_ESPRegenFault_flg/2  "<VSRV_ESPRegenFaultIn_flg_ovrdflg>"
  Bus Selector14/1 -> Subsys VINP_ESPRegenFault_flg/3  "<VSRV_ESPRegenFaultIn_flg_ovrdval>"
  [MsgAlive_flgs] -> Subsys VINP_ESPRegenFault_flg/4
  Subsys VINP_ESPRegenFault_flg/1 -> Bus Creator/2  "VINP_ESPRegenFault_flg"
  Subsys VINP_ESPRegenFault_flg/2 -> Terminator1/1
  Bus Selector16/1 -> Subsys VINP_ESPRegenTargetAtWheel_Nm/1  "<VHAL_ESPRegenTargetAtWheelIn_Nm>"
  Bus Selector4/1 -> Subsys VINP_ESPRegenTargetAtWheel_Nm/2  "<VHAL_ESPRegenTargetValidIn_flg>"
  Bus Selector18/1 -> Subsys VINP_ESPRegenTargetAtWheel_Nm/3  "<VSRV_ESPRegenTargetIn_Nm_ovrdflg>"
  Bus Selector15/1 -> Subsys VINP_ESPRegenTargetAtWheel_Nm/4  "<VSRV_ESPRegenTargetIn_Nm_ovrdval>"
  [MsgAlive_flgs] -> Subsys VINP_ESPRegenTargetAtWheel_Nm/5
  Subsys VINP_ESPRegenTargetAtWheel_Nm/1 -> Bus Creator/3  "VINP_ESPRegenTargetAtWheel_Nm"
  Subsys VINP_ESPRegenTargetAtWheel_Nm/2 -> Terminator2/1

== system inp/INP/INP_20MS/Message (20ms) EMS_HSC_FrP01 ==
  BHAL_IN_20ms : Inport
  BSRV_In_ovrdflgs : Inport  Port=2
  BSRV_In_ovrdvals : Inport  Port=3
  VINP_EMSMsgAlive_flg : Inport  Port=4
  Bus Creator : BusCreator  Inputs=5
  Bus Selector11 : BusSelector  OutputSignals=VHAL_CruiseControlActiveIn_flg
  Bus Selector13 : BusSelector  OutputSignals=VSRV_CruiseControlActiveIn_flg_ovrdflg
  Bus Selector14 : BusSelector  OutputSignals=VSRV_CruiseControlActiveIn_flg_ovrdval
  Bus Selector2 : BusSelector  OutputSignals=VSRV_EMSHSCFrP01Active_flg_ovrdflg
  Bus Selector3 : BusSelector  OutputSignals=VSRV_EMSHSCFrP01Active_flg_ovrdval
  Bus Selector34 : BusSelector  OutputSignals=VHAL_EngCoolantTempIn_C,VHAL_EngCoolantTempValidIn_flg
  Bus Selector36 : BusSelector  OutputSignals=VSRV_EngCoolantTempIn_C_ovrdflg
  Bus Selector4 : BusSelector  OutputSignals=VSRV_EngCoolantTempIn_C_ovrdval
  Bus Selector55 : BusSelector  OutputSignals=VHAL_EngIdleTypeReqIn_enum
  Bus Selector57 : BusSelector  OutputSignals=VSRV_EngIdleTypeReqIn_enum_ovrdflg
  Bus Selector58 : BusSelector  OutputSignals=VSRV_EngIdleTypeReqIn_enum_ovrdval
  Subsys VINP_CruiseControlActive_flg : inp_lib/msgactv_ovrd  SystemSampleTime=-1  cal_ovrdflg=KINP_CruiseControlActive_flg_ovrdflg  cal_ovrdval=KINP_CruiseControlActive_flg_ovrdval  default=KINP_CruiseControlActiveDefault_flg
  Subsys VINP_EMSHSCFrP01Active_flg : inp_lib/override  SystemSampleTime=-1  cal_ovrdflg=KINP_EMSHSCFrP01Active_ovrdflg  cal_ovrdval=KINP_EMSHSCFrP01Active_flg_ovrdval
  Subsys VINP_EngCoolantTemp_C : inp_lib/valid_msgactv_sat_ovrd  SystemSampleTime=-1  cal_ovrdflg=KINP_EngCoolantTemp_C_ovrdflg  cal_ovrdval=KINP_EngCoolantTemp_C_ovrdval  lim=KINP_ValidCheck_EngCoolantTemp_lim  inc=KINP_ValidCheck_EngCoolantTemp_inc  dec=KINP_ValidCheck_EngCoolantTemp_dec  default=KINP_EngCoolantTempDefault_C  hi=KINP_EngCoolantTemp_C_Max  lo=KINP_EngCoolantTemp_C_Min
  Subsys VINP_EngIdleTypeReq_enum : inp_lib/msgactv_sat_ovrd  SystemSampleTime=-1  cal_ovrdflg=KINP_EngIdleTypeReq_enum_ovrdflg  cal_ovrdval=KINP_EngIdleTypeReq_enum_ovrdval  default=KINP_EngIdleTypeReqDefault_enum  hi=KINP_EngIdleTypeReq_enum_Max  lo=KINP_EngIdleTypeReq_enum_Min
  Terminator : Terminator
  Terminator1 : Terminator
  BINP_EMS_HSC_FrP01 : Outport
  wires:
  [VINP_EMSMsgAlive_flg] -> [MsgAlive_flgs], Subsys VINP_EMSHSCFrP01Active_flg/1
  [BSRV_In_ovrdflgs] -> Bus Selector2/1
  [BSRV_In_ovrdvals] -> Bus Selector3/1
  [BSRV_In_ovrdvals] -> Bus Selector14/1
  [BSRV_In_ovrdflgs] -> Bus Selector13/1
  [BSRV_In_ovrdflgs] -> Bus Selector57/1
  [BSRV_In_ovrdvals] -> Bus Selector58/1
  BHAL_IN_20ms/1 -> Bus Selector11/1, Bus Selector55/1, Bus Selector34/1
  [BSRV_In_ovrdvals] -> Bus Selector4/1
  [BSRV_In_ovrdflgs] -> Bus Selector36/1
  VINP_EMSMsgAlive_flg/1 -> [VINP_EMSMsgAlive_flg]
  BSRV_In_ovrdflgs/1 -> [BSRV_In_ovrdflgs]
  BSRV_In_ovrdvals/1 -> [BSRV_In_ovrdvals]
  Bus Creator/1 -> BINP_EMS_HSC_FrP01/1  "BINP_EMS_HSC_FrP01"
  Bus Selector11/1 -> Subsys VINP_CruiseControlActive_flg/1  "<VHAL_CruiseControlActiveIn_flg>"
  Bus Selector13/1 -> Subsys VINP_CruiseControlActive_flg/2  "<VSRV_CruiseControlActiveIn_flg_ovrdflg>"
  Bus Selector14/1 -> Subsys VINP_CruiseControlActive_flg/3  "<VSRV_CruiseControlActiveIn_flg_ovrdval>"
  [MsgAlive_flgs] -> Subsys VINP_CruiseControlActive_flg/4
  Subsys VINP_CruiseControlActive_flg/1 -> Bus Creator/4  "VINP_CruiseControlActive_flg"
  Subsys VINP_CruiseControlActive_flg/2 -> Terminator/1
  Bus Selector2/1 -> Subsys VINP_EMSHSCFrP01Active_flg/2  "<VSRV_EMSHSCFrP01Active_flg_ovrdflg>"
  Bus Selector3/1 -> Subsys VINP_EMSHSCFrP01Active_flg/3  "<VSRV_EMSHSCFrP01Active_flg_ovrdval>"
  Subsys VINP_EMSHSCFrP01Active_flg/1 -> Bus Creator/5  "VINP_EMSHSCFrP01Active_flg"
  Bus Selector34/1 -> Subsys VINP_EngCoolantTemp_C/1  "<VHAL_EngCoolantTempIn_C>"
  Bus Selector34/2 -> Subsys VINP_EngCoolantTemp_C/2  "<VHAL_EngCoolantTempValidIn_flg>"
  Bus Selector36/1 -> Subsys VINP_EngCoolantTemp_C/3  "<VSRV_EngCoolantTempIn_C_ovrdflg>"
  Bus Selector4/1 -> Subsys VINP_EngCoolantTemp_C/4  "<VSRV_EngCoolantTempIn_C_ovrdval>"
  [MsgAlive_flgs] -> Subsys VINP_EngCoolantTemp_C/5
  Subsys VINP_EngCoolantTemp_C/1 -> Bus Creator/1  "VINP_EngCoolantTemp_C"
  Subsys VINP_EngCoolantTemp_C/2 -> Bus Creator/2  "VINP_EngCoolantTempValid_flg"
  Bus Selector55/1 -> Subsys VINP_EngIdleTypeReq_enum/1  "<VHAL_EngIdleTypeReqIn_enum>"
  Bus Selector57/1 -> Subsys VINP_EngIdleTypeReq_enum/2  "<VSRV_EngIdleTypeReqIn_enum_ovrdflg>"
  Bus Selector58/1 -> Subsys VINP_EngIdleTypeReq_enum/3  "<VSRV_EngIdleTypeReqIn_enum_ovrdval>"
  [MsgAlive_flgs] -> Subsys VINP_EngIdleTypeReq_enum/4
  Subsys VINP_EngIdleTypeReq_enum/1 -> Bus Creator/3  "VINP_EngIdleTypeReq_enum"
  Subsys VINP_EngIdleTypeReq_enum/2 -> Terminator1/1

== system inp/INP/INP_20MS/Message (20ms) EPB_HSC_FrP00 ==
  BHAL_IN_20ms : Inport
  BSRV_In_ovrdflgs : Inport  Port=2
  BSRV_In_ovrdvals : Inport  Port=3
  VINP_EPBMsgAlive_flg : Inport  Port=4
  Bus Creator1 : BusCreator  Inputs=3
  Bus Selector3 : BusSelector  OutputSignals=VSRV_EPBHSCFrP00Active_flg_ovrdval
  Bus Selector37 : BusSelector  OutputSignals=VSRV_GSensorIn_g_ovrdflg
  Bus Selector38 : BusSelector  OutputSignals=VSRV_GSensorIn_g_ovrdval
  Bus Selector39 : BusSelector  OutputSignals=VHAL_GSensorIn_g
  Bus Selector4 : BusSelector  OutputSignals=VSRV_EPBHSCFrP00Active_flg_ovrdflg
  Bus Selector55 : BusSelector  OutputSignals=VHAL_EPBStatusIn_enum
  Bus Selector57 : BusSelector  OutputSignals=VSRV_EPBStatusIn_enum_ovrdflg
  Bus Selector58 : BusSelector  OutputSignals=VSRV_EPBStatusIn_enum_ovrdval
  Subsys VINP_EPBHSCFrP00Active_flg : inp_lib/override  SystemSampleTime=-1  cal_ovrdflg=KINP_EPBHSCFrP00Active_ovrdflg  cal_ovrdval=KINP_EPBHSCFrP00Active_flg_ovrdval
  Subsys VINP_EPBStatus_enum : inp_lib/msgactv_sat_ovrd  SystemSampleTime=-1  cal_ovrdflg=KINP_EPBStatus_enum_ovrdflg  cal_ovrdval=KINP_EPBStatus_enum_ovrdval  default=KINP_EPBStatusDefault_enum  hi=KINP_EPBStatus_enum_Max  lo=KINP_EPBStatus_enum_Min
  Subsys VINP_GSensor_g : inp_lib/msgactv_sat_ovrd  SystemSampleTime=-1  cal_ovrdflg=KINP_GSensor_g_ovrdflg  cal_ovrdval=KINP_GSensor_g_ovrdval  default=KINP_GSensorDefault_g  hi=KINP_GSensor_g_Max  lo=KINP_GSensor_g_Min
  Terminator : Terminator
  Terminator1 : Terminator
  BINP_EPB_HSC_FrP00 : Outport
  wires:
  Bus Creator1/1 -> BINP_EPB_HSC_FrP00/1  "BINP_EPB_HSC_FrP00"
  BSRV_In_ovrdvals/1 -> [BSRV_In_ovrdvals]
  BSRV_In_ovrdflgs/1 -> [BSRV_In_ovrdflgs]
  VINP_EPBMsgAlive_flg/1 -> [VINP_EPBMsgAlive_flg]
  BHAL_IN_20ms/1 -> Bus Selector39/1, Bus Selector55/1
  [BSRV_In_ovrdvals] -> Bus Selector38/1
  [BSRV_In_ovrdflgs] -> Bus Selector37/1
  [BSRV_In_ovrdflgs] -> Bus Selector57/1
  [BSRV_In_ovrdvals] -> Bus Selector58/1
  [VINP_EPBMsgAlive_flg] -> [MsgAlive_flgs], Subsys VINP_EPBHSCFrP00Active_flg/1  "VHAL_EPBHSCFrP00Active_flg"
  [BSRV_In_ovrdflgs] -> Bus Selector4/1
  [BSRV_In_ovrdvals] -> Bus Selector3/1
  Bus Selector4/1 -> Subsys VINP_EPBHSCFrP00Active_flg/2  "<VSRV_EPBHSCFrP00Active_flg_ovrdflg>"
  Bus Selector3/1 -> Subsys VINP_EPBHSCFrP00Active_flg/3  "<VSRV_EPBHSCFrP00Active_flg_ovrdval>"
  Subsys VINP_EPBHSCFrP00Active_flg/1 -> Bus Creator1/3  "VINP_EPBHSCFrP00Active_flg"
  Bus Selector55/1 -> Subsys VINP_EPBStatus_enum/1  "<VHAL_EPBStatusIn_enum>"
  Bus Selector57/1 -> Subsys VINP_EPBStatus_enum/2  "<VSRV_EPBStatusIn_enum_ovrdflg>"
  Bus Selector58/1 -> Subsys VINP_EPBStatus_enum/3  "<VSRV_EPBStatusIn_enum_ovrdval>"
  [MsgAlive_flgs] -> Subsys VINP_EPBStatus_enum/4
  Subsys VINP_EPBStatus_enum/1 -> Bus Creator1/2  "VINP_EPBStatus_enum"
  Subsys VINP_EPBStatus_enum/2 -> Terminator/1
  Bus Selector39/1 -> Subsys VINP_GSensor_g/1  "<VHAL_GSensorIn_g>"
  Bus Selector37/1 -> Subsys VINP_GSensor_g/2  "<VSRV_GSensorIn_g_ovrdflg>"
  Bus Selector38/1 -> Subsys VINP_GSensor_g/3  "<VSRV_GSensorIn_g_ovrdval>"
  [MsgAlive_flgs] -> Subsys VINP_GSensor_g/4
  Subsys VINP_GSensor_g/1 -> Bus Creator1/1  "VINP_GSensor_g"
  Subsys VINP_GSensor_g/2 -> Terminator1/1

== system inp/INP/INP_20MS/Message (20ms) SMU_HSC_FrP02 ==
  BHAL_IN_20ms : Inport
  BSRV_In_ovrdflgs : Inport  Port=2
  BSRV_In_ovrdvals : Inport  Port=3
  VINP_SMUMsgAlive_flg : Inport  Port=4
  Bus Creator : BusCreator  Inputs=2
  Bus Selector1 : BusSelector  OutputSignals=VSRV_SMUHSCFrP02Active_flg_ovrdval
  Bus Selector11 : BusSelector  OutputSignals=VSRV_SecurityKeyValidIn_flg_ovrdval
  Bus Selector2 : BusSelector  OutputSignals=VSRV_SMUHSCFrP02Active_flg_ovrdflg
  Bus Selector3 : BusSelector  OutputSignals=VHAL_SecurityKeyValidIn_flg
  Bus Selector6 : BusSelector  OutputSignals=VSRV_SecurityKeyValidIn_flg_ovrdflg
  Subsys VINP_SMUHSCFrP02Active_flg : inp_lib/override  SystemSampleTime=-1  cal_ovrdflg=KINP_SMUHSCFrP02Active_ovrdflg  cal_ovrdval=KINP_SMUHSCFrP02Active_flg_ovrdval
  Subsys VINP_SecurityKeyValid_flg : inp_lib/msgactv_ovrd  SystemSampleTime=-1  cal_ovrdflg=KINP_SecurityKeyValid_flg_ovrdflg  cal_ovrdval=KINP_SecurityKeyValid_flg_ovrdval  default=KINP_SecurityKeyValidDefault_flg
  Terminator : Terminator
  BINP_SMU_HSC_FrP02 : Outport
  wires:
  BHAL_IN_20ms/1 -> Bus Selector3/1
  [BSRV_In_ovrdvals] -> Bus Selector11/1
  [BSRV_In_ovrdflgs] -> Bus Selector6/1
  VINP_SMUMsgAlive_flg/1 -> [VINP_SMUMsgAlive_flg]
  BSRV_In_ovrdflgs/1 -> [BSRV_In_ovrdflgs]
  BSRV_In_ovrdvals/1 -> [BSRV_In_ovrdvals]
  Bus Creator/1 -> BINP_SMU_HSC_FrP02/1  "BINP_SMU_HSC_FrP02"
  [VINP_SMUMsgAlive_flg] -> [MsgAlive_flgs], Subsys VINP_SMUHSCFrP02Active_flg/1
  [BSRV_In_ovrdflgs] -> Bus Selector2/1
  [BSRV_In_ovrdvals] -> Bus Selector1/1
  Bus Selector2/1 -> Subsys VINP_SMUHSCFrP02Active_flg/2  "<VSRV_SMUHSCFrP02Active_flg_ovrdflg>"
  Bus Selector1/1 -> Subsys VINP_SMUHSCFrP02Active_flg/3  "<VSRV_SMUHSCFrP02Active_flg_ovrdval>"
  Subsys VINP_SMUHSCFrP02Active_flg/1 -> Bus Creator/2  "VINP_SMUHSCFrP02Active_flg"
  Bus Selector3/1 -> Subsys VINP_SecurityKeyValid_flg/1  "<VHAL_SecurityKeyValidIn_flg>"
  Bus Selector6/1 -> Subsys VINP_SecurityKeyValid_flg/2  "<VSRV_SecurityKeyValidIn_flg_ovrdflg>"
  Bus Selector11/1 -> Subsys VINP_SecurityKeyValid_flg/3  "<VSRV_SecurityKeyValidIn_flg_ovrdval>"
  [MsgAlive_flgs] -> Subsys VINP_SecurityKeyValid_flg/4
  Subsys VINP_SecurityKeyValid_flg/1 -> Bus Creator/1  "VINP_SecurityKeyValid_flg"
  Subsys VINP_SecurityKeyValid_flg/2 -> Terminator/1

== system inp/INP/INP_50MS/BSRV_In_ovrdflgs ==
  Constant: VSRV_AmbientTempIn_C_ovrdflg : Constant  Value=0  OutDataTypeMode=boolean  OutDataTypeStr=boolean
  Constant: VSRV_AmbientTempValidIn_flg_ovrdflg : Constant  Value=0  OutDataTypeMode=boolean  OutDataTypeStr=boolean
  Constant: VSRV_BMSCellTempMinIn_C_ovrdflg : Constant  Value=0  OutDataTypeMode=boolean  OutDataTypeStr=boolean
  Constant: VSRV_BMSCellTempMinValidIn_C_ovrdflg : Constant  Value=0  OutDataTypeMode=boolean  OutDataTypeStr=boolean
  Constant: VSRV_BMSColdCrkCtrlIn_enum_ovrdflg : Constant  Value=0  OutDataTypeMode=boolean  OutDataTypeStr=boolean
  Constant: VSRV_BMSHSC2FrP01Active_flg_ovrdflg : Constant  Value=0  OutDataTypeMode=boolean  OutDataTypeStr=boolean
  Constant: VSRV_BMSHSC2FrP01ProtFault_flg_ovrdflg : Constant  Value=0  OutDataTypeMode=boolean  OutDataTypeStr=boolean
  Constant: VSRV_BMSHSC2FrP02Active_flg_ovrdflg : Constant  Value=0  OutDataTypeMode=boolean  OutDataTypeStr=boolean
  Constant: VSRV_BMSHSC2FrP02ProtFault_flg_ovrdflg : Constant  Value=0  OutDataTypeMode=boolean  OutDataTypeStr=boolean
  Constant: VSRV_BMSMainRelayStatIn_enum_ovrdflg : Constant  Value=0  OutDataTypeMode=boolean  OutDataTypeStr=boolean
  Constant: VSRV_BMSPackSOCDispIn_pct_ovrdflg : Constant  Value=0  OutDataTypeMode=boolean  OutDataTypeStr=boolean
  Constant: VSRV_BMSPackSOCDispValidIn_pct_ovrdflg : Constant  Value=0  OutDataTypeMode=boolean  OutDataTypeStr=boolean
  Constant: VSRV_HVBattBasicStatusIn_enum_ovrdflg : Constant  Value=0  OutDataTypeMode=boolean  OutDataTypeStr=boolean
  Constant: VSRV_HVBattCellTempMaxIn_C_ovrdflg : Constant  Value=0  OutDataTypeMode=boolean  OutDataTypeStr=boolean
  Constant: VSRV_HVBattCellTempMaxValidIn_flg_ovrdflg : Constant  Value=0  OutDataTypeMode=boolean  OutDataTypeStr=boolean
  Constant: VSRV_HVBattChargerPluggedIn_flg_ovrdflg : Constant  Value=0  OutDataTypeMode=boolean  OutDataTypeStr=boolean
  Constant: VSRV_HVBattChillerOffReqIn_flg_ovrdflg : Constant  Value=0  OutDataTypeMode=boolean  OutDataTypeStr=boolean
  Constant: VSRV_HVBattCoolantTempIn_C_ovrdflg : Constant  Value=0  OutDataTypeMode=boolean  OutDataTypeStr=boolean
  Constant: VSRV_HVBattCoolantTempValidIn_flg_ovrdflg : Constant  Value=0  OutDataTypeMode=boolean  OutDataTypeStr=boolean
  Constant: VSRV_HVBattCoolingPumpStatusIn_enum_ovrdflg : Constant  Value=0  OutDataTypeMode=boolean  OutDataTypeStr=boolean
  Constant: VSRV_HVBattCurrentIn_A_ovrdflg : Constant  Value=0  OutDataTypeMode=boolean  OutDataTypeStr=boolean
  Constant: VSRV_HVBattCurrentValidIn_flg_ovrdflg : Constant  Value=0  OutDataTypeMode=boolean  OutDataTypeStr=boolean
  Constant: VSRV_HVBattHVILClosedIn_flg_ovrdflg : Constant  Value=0  OutDataTypeMode=boolean  OutDataTypeStr=boolean
  Constant: VSRV_HVBattIsolationResistanceIn_kohm_ovrdflg : Constant  Value=0  OutDataTypeMode=boolean  OutDataTypeStr=boolean
  Constant: VSRV_HVBattIsolationResistanceValidIn_flg_ovrdflg : Constant  Value=0  OutDataTypeMode=boolean  OutDataTypeStr=boolean
  Constant: VSRV_HVBattSOCIn_pct_ovrdflg : Constant  Value=0  OutDataTypeMode=boolean  OutDataTypeStr=boolean
  Constant: VSRV_HVBattSOCValidIn_flg_ovrdflg : Constant  Value=0  OutDataTypeMode=boolean  OutDataTypeStr=boolean
  Constant: VSRV_HVBattVoltageIn_V_ovrdflg : Constant  Value=0  OutDataTypeMode=boolean  OutDataTypeStr=boolean
  Constant: VSRV_HVBattVoltageValidIn_flg_ovrdflg : Constant  Value=0  OutDataTypeMode=boolean  OutDataTypeStr=boolean
  Constant: VSRV_KeySwitchStateCRKIn_flg_ovrdflg : Constant  Value=0  OutDataTypeMode=boolean  OutDataTypeStr=boolean
  Constant: VSRV_SMUHSCFrP00Active_flg_ovrdflg : Constant  Value=0  OutDataTypeMode=boolean  OutDataTypeStr=boolean
  Constant: VSRV_SMUHSCFrP03Active_flg_ovrdflg : Constant  Value=0  OutDataTypeMode=boolean  OutDataTypeStr=boolean
  Constant: VSRV_SMUHSCFrP08Active_flg_ovrdflg : Constant  Value=0  OutDataTypeMode=boolean  OutDataTypeStr=boolean
  inputs_bus : BusCreator  Inputs=33
  output_bus : Outport
  wires:
  Constant: VSRV_BMSPackSOCDispValidIn_pct_ovrdflg/1 -> inputs_bus/33  "VSRV_BMSPackSOCDispValidIn_pct_ovrdflg"
  Constant: VSRV_BMSPackSOCDispIn_pct_ovrdflg/1 -> inputs_bus/32  "VSRV_BMSPackSOCDispIn_pct_ovrdflg"
  Constant: VSRV_BMSCellTempMinValidIn_C_ovrdflg/1 -> inputs_bus/31  "VSRV_BMSCellTempMinValidIn_C_ovrdflg"
  Constant: VSRV_BMSCellTempMinIn_C_ovrdflg/1 -> inputs_bus/30  "VSRV_BMSCellTempMinIn_C_ovrdflg"
  Constant: VSRV_BMSColdCrkCtrlIn_enum_ovrdflg/1 -> inputs_bus/29  "VSRV_BMSColdCrkCtrlIn_enum_ovrdflg"
  Constant: VSRV_SMUHSCFrP00Active_flg_ovrdflg/1 -> inputs_bus/28  "VSRV_SMUHSCFrP00Active_flg_ovrdflg"
  Constant: VSRV_HVBattIsolationResistanceValidIn_flg_ovrdflg/1 -> inputs_bus/27  "VSRV_HVBattIsolationResistanceValidIn_flg_ovrdflg"
  Constant: VSRV_HVBattIsolationResistanceIn_kohm_ovrdflg/1 -> inputs_bus/26  "VSRV_HVBattIsolationResistanceIn_kohm_ovrdflg"
  Constant: VSRV_SMUHSCFrP08Active_flg_ovrdflg/1 -> inputs_bus/25  "VSRV_SMUHSCFrP08Active_flg_ovrdflg"
  Constant: VSRV_SMUHSCFrP03Active_flg_ovrdflg/1 -> inputs_bus/24  "VSRV_SMUHSCFrP03Active_flg_ovrdflg"
  Constant: VSRV_KeySwitchStateCRKIn_flg_ovrdflg/1 -> inputs_bus/23  "VSRV_KeySwitchStateCRKIn_flg_ovrdflg"
  Constant: VSRV_HVBattVoltageValidIn_flg_ovrdflg/1 -> inputs_bus/22  "VSRV_HVBattVoltageValidIn_flg_ovrdflg"
  Constant: VSRV_HVBattVoltageIn_V_ovrdflg/1 -> inputs_bus/21  "VSRV_HVBattVoltageIn_V_ovrdflg"
  Constant: VSRV_HVBattSOCValidIn_flg_ovrdflg/1 -> inputs_bus/20  "VSRV_HVBattSOCValidIn_flg_ovrdflg"
  Constant: VSRV_HVBattSOCIn_pct_ovrdflg/1 -> inputs_bus/19  "VSRV_HVBattSOCIn_pct_ovrdflg"
  Constant: VSRV_HVBattBasicStatusIn_enum_ovrdflg/1 -> inputs_bus/18  "VSRV_HVBattBasicStatusIn_enum_ovrdflg"
  Constant: VSRV_HVBattHVILClosedIn_flg_ovrdflg/1 -> inputs_bus/17  "VSRV_HVBattHVILClosedIn_flg_ovrdflg"
  Constant: VSRV_HVBattCurrentValidIn_flg_ovrdflg/1 -> inputs_bus/16  "VSRV_HVBattCurrentValidIn_flg_ovrdflg"
  Constant: VSRV_HVBattCurrentIn_A_ovrdflg/1 -> inputs_bus/15  "VSRV_HVBattCurrentIn_A_ovrdflg"
  Constant: VSRV_HVBattCoolingPumpStatusIn_enum_ovrdflg/1 -> inputs_bus/14  "VSRV_HVBattCoolingPumpStatusIn_enum_ovrdflg"
  Constant: VSRV_HVBattCoolantTempValidIn_flg_ovrdflg/1 -> inputs_bus/13  "VSRV_HVBattCoolantTempValidIn_flg_ovrdflg"
  Constant: VSRV_HVBattCoolantTempIn_C_ovrdflg/1 -> inputs_bus/12  "VSRV_HVBattCoolantTempIn_C_ovrdflg"
  Constant: VSRV_HVBattChillerOffReqIn_flg_ovrdflg/1 -> inputs_bus/11  "VSRV_HVBattChillerOffReqIn_flg_ovrdflg"
  Constant: VSRV_HVBattChargerPluggedIn_flg_ovrdflg/1 -> inputs_bus/10  "VSRV_HVBattChargerPluggedIn_flg_ovrdflg"
  Constant: VSRV_HVBattCellTempMaxValidIn_flg_ovrdflg/1 -> inputs_bus/9  "VSRV_HVBattCellTempMaxValidIn_flg_ovrdflg"
  Constant: VSRV_HVBattCellTempMaxIn_C_ovrdflg/1 -> inputs_bus/8  "VSRV_HVBattCellTempMaxIn_C_ovrdflg"
  Constant: VSRV_BMSMainRelayStatIn_enum_ovrdflg/1 -> inputs_bus/7  "VSRV_BMSMainRelayStatIn_enum_ovrdflg"
  Constant: VSRV_BMSHSC2FrP02Active_flg_ovrdflg/1 -> inputs_bus/6  "VSRV_BMSHSC2FrP02Active_flg_ovrdflg"
  Constant: VSRV_BMSHSC2FrP01Active_flg_ovrdflg/1 -> inputs_bus/5  "VSRV_BMSHSC2FrP01Active_flg_ovrdflg"
  Constant: VSRV_AmbientTempValidIn_flg_ovrdflg/1 -> inputs_bus/4  "VSRV_AmbientTempValidIn_flg_ovrdflg"
  Constant: VSRV_AmbientTempIn_C_ovrdflg/1 -> inputs_bus/3  "VSRV_AmbientTempIn_C_ovrdflg"
  Constant: VSRV_BMSHSC2FrP02ProtFault_flg_ovrdflg/1 -> inputs_bus/2  "VSRV_BMSHSC2FrP02ProtFault_flg_ovrdflg"
  Constant: VSRV_BMSHSC2FrP01ProtFault_flg_ovrdflg/1 -> inputs_bus/1  "VSRV_BMSHSC2FrP01ProtFault_flg_ovrdflg"
  inputs_bus/1 -> output_bus/1  "output_bus"
